simulink model "ycoilSintonization"  (R2024a)
settings: Solver=VariableStepAuto  StartTime=0.0  StopTime=1000  RelTol=1e-3
values from neighbouring files (symbols this model uses):
  y = yout(:,2)    [myObjectiveFunction.m]
libraries: simulink x1
settings Model: Creator=b_ant  LastModifiedBy=b_ant
settings DataIOCC: SaveFormat=Array

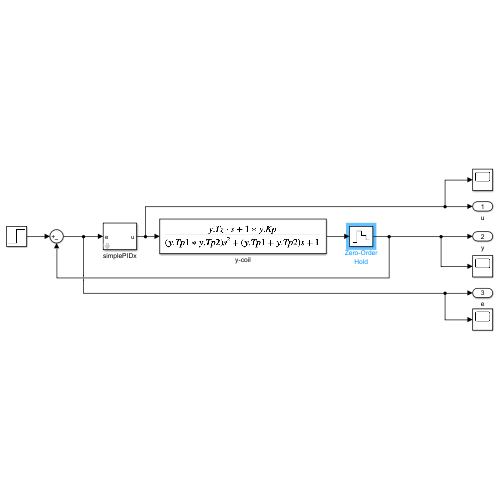
[thumbnail: Simulink's stored preview of the top-level diagram]
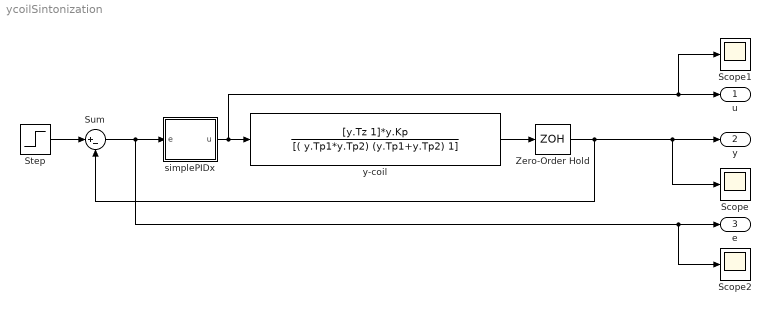
== system ycoilSintonization ==
  Scope : Scope
  Scope1 : Scope
  Scope2 : Scope
  Step : Step  Time=0.001  SampleTime=0
  Sum : Sum  Inputs=|+-
  Zero-Order Hold : ZeroOrderHold
  simplePIDx : Subsystem  mask{Gain1=y.PID.Kd, Gain2=y.PID.Ki, Gain3=y.PID.Kp}
      mask prompts: Gain1 "kd:"; Gain2 "ki:"; Gain3 "kp:"
      mask TypeOptions Gain1: PID kd/Gain
      mask TypeOptions Gain2: PID ki/Gain
      mask TypeOptions Gain3: PID kp/Gain
  y-coil : TransferFcn  Numerator=[y.Tz 1]*y.Kp  Denominator=[( y.Tp1*y.Tp2) (y.Tp1+y.Tp2) 1]
  u : Outport
  y : Outport  Port=2
  e : Outport  Port=3
  wires:
  Zero-Order Hold/1 -> Scope/1, y/1, Sum/2
  y-coil/1 -> Zero-Order Hold/1
  Sum/1 -> simplePIDx/1(e), Scope2/1, e/1
  simplePIDx/1(u) -> y-coil/1, Scope1/1, u/1
  Step/1 -> Sum/1

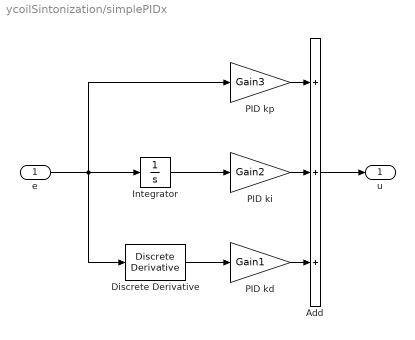
== system ycoilSintonization/simplePIDx ==
  e : Inport
  Add : Sum  Inputs=+++
  Discrete Derivative : simulink/Discrete/Discrete Derivative  gainval=1.0  ICPrevScaledInput=0.0  OutMin=[]  OutMax=[]  OutDataType=fixdt(1, 16)  OutScaling=2^-10  DoSatur=off
  Integrator : Integrator
  PID kd : Gain  Gain=Gain1
  PID ki : Gain  Gain=Gain2
  PID kp : Gain  Gain=Gain3
  u : Outport
  wires:
  Discrete Derivative/1 -> PID kd/1
  Add/1 -> u/1
  e/1 -> PID kp/1, Integrator/1, Discrete Derivative/1
  Integrator/1 -> PID ki/1
  PID ki/1 -> Add/2
  PID kd/1 -> Add/3
  PID kp/1 -> Add/1
